simulink model "Xcvr_SSB_AM_2p5"  (Simulink 7.4)
settings: Solver=VariableStepDiscrete  SolverMode=SingleTasking  StartTime=0.0  StopTime=10  RelTol=1e-3
PreLoadFcn:
  | Fs=80e6;
  | 
  | phee=da_rom();
  | [phee_1,phee_2]=da_i2_rom();
  | 
  | Dcic=64;       % CIC decimation
  | Dfac=128;    % following DA filter decimation
  | N = 6;           %       (2^(N+1))=Dfac
  | Daudio=Dcic*Dfac;
  | Faudio=Fs/Daudio;
  | 
  | load info_filt_ssb_4
  | load Serial_Intfc_Stream_5
  | 
  | % AGC related
  | x=0.5:1/256:(1-1/256);
  | addr=(x-0.5)*256;
  | y=1./x;
undefined symbols (not defined in the file): Serial_Interface, ssb_coef, xlipgetpartsetting
libraries: xbsIndex_r4 x1305, dspsrcs4 x5, simulink x2, dspsigops x2, dspsnks4 x1
(part 8 of 11)

== system Xcvr_SSB_AM_2p5/TX Filters I=8192/Interp_Core/ROM/Accumulator ==
  Xn + Xn-4 : Inport
  "Xn-1+ Xn-3 " : Inport  Port=2
  Xn-2 : Inport  Port=3
  Yn-1 : Inport  Port=4
  Yn-2 : Inport  Port=5
  Xn+Xn-3 : Inport  Port=6
  Xn-1+Xn-2 : Inport  Port=7
  Zn-1 : Inport  Port=8
  Zn-2 : Inport  Port=9
  Round : Inport  Port=10
  Clear Acc : Inport  Port=11
  Subtract : Inport  Port=12
  AddSub{,1..3} (4 alike) : xbsIndex_r4/AddSub  mode=Addition  use_carryin=off  use_carryout=off  en=off  latency=0  precision=User Defined  arith_type="Signed  (2's comp)"  n_bits=18+1  bin_pt=0  quantization=Truncate  overflow=Wrap  dbl_ovrd=off  use_behavioral_HDL=off  hw_selection=Fabric  pipelined=off  use_rpm=on  block_type=addsub
      settings: block_version=9.2.00
  Concat : xbsIndex_r4/Concat  num_inputs=6  dbl_ovrd=off  block_type=concat
      settings: block_version=9.2.00
  Concat1 : xbsIndex_r4/Concat  num_inputs=5  dbl_ovrd=off  block_type=concat
      settings: block_version=9.2.00
  Convert : xbsIndex_r4/Convert  arith_type="Signed  (2's comp)"  n_bits=2  bin_pt=0  quantization=Truncate  overflow=Wrap  en=off  latency=0  dbl_ovrd=off  pipeline=off  block_type=convert
      settings: block_version=9.2.00
  Phee_1 ROM : xbsIndex_r4/ROM  depth=64  initVector=phee_1  distributed_mem=Block RAM  rst=off  init_reg=0  en=off  latency=1  arith_type="Signed  (2's comp)"  n_bits=13  bin_pt=0  dbl_ovrd=off  optimize=Area  use_rpm=on  block_type=sprom
      settings: block_version=9.2.00
  Phee_2 ROM : xbsIndex_r4/ROM  depth=32  initVector=phee_2  distributed_mem=Block RAM  rst=off  init_reg=0  en=off  latency=1  arith_type="Signed  (2's comp)"  n_bits=13  bin_pt=0  dbl_ovrd=off  optimize=Area  use_rpm=on  block_type=sprom
      settings: block_version=9.2.00
  Register1 : xbsIndex_r4/Register  init=0  rst=on  en=off  dbl_ovrd=off  block_type=register
      settings: block_version=9.2.00
  Register2 : xbsIndex_r4/Register  init=0  rst=on  en=off  dbl_ovrd=off  block_type=register
      settings: block_version=9.2.00
  Reinterpret1 : xbsIndex_r4/Reinterpret  force_arith_type=on  arith_type="Signed  (2's comp)"  force_bin_pt=on  bin_pt=0  block_type=reinterpret
      settings: infoedit="Changes signal type without altering the binary representation.   You can changed the signal between signed and unsigned, and relocate the binary point.<P><P>Hardware notes: In hardware this block costs nothing.<P><P>Example:  Suppose the input is 6 bits wide, signed, with 2 fractional bits, and the output is forced to unsigned with 0 fractional bits.  Then an input of -2.0 (1110.00 in binary 2's complement) becomes an output of 56 (111000 in binary)."  block_version=9.2.00
  Reinterpret2 : xbsIndex_r4/Reinterpret  force_arith_type=on  arith_type="Signed  (2's comp)"  force_bin_pt=on  bin_pt=0  block_type=reinterpret
      settings: infoedit="Changes signal type without altering the binary representation.   You can changed the signal between signed and unsigned, and relocate the binary point.<P><P>Hardware notes: In hardware this block costs nothing.<P><P>Example:  Suppose the input is 6 bits wide, signed, with 2 fractional bits, and the output is forced to unsigned with 0 fractional bits.  Then an input of -2.0 (1110.00 in binary 2's complement) becomes an output of 56 (111000 in binary)."  block_version=9.2.00
  Shift1 : xbsIndex_r4/Shift  shift_dir=Left  shift_bits=5  en=off  latency=0  precision=User Defined  arith_type="Signed  (2's comp)"  n_bits=18  bin_pt=0  quantization=Truncate  overflow=Wrap  dbl_ovrd=off  block_type=shift
      settings: block_version=9.2.00
  Shift2 : xbsIndex_r4/Shift  shift_dir=Left  shift_bits=5  en=off  latency=0  precision=User Defined  arith_type="Signed  (2's comp)"  n_bits=18  bin_pt=0  quantization=Truncate  overflow=Wrap  dbl_ovrd=off  block_type=shift
      settings: block_version=9.2.00
  Shift3 : xbsIndex_r4/Shift  shift_dir=Right  shift_bits=1  en=off  latency=0  precision=Full  arith_type="Signed  (2's comp)"  n_bits=18  bin_pt=0  quantization=Truncate  overflow=Wrap  dbl_ovrd=off  block_type=shift
      settings: block_version=9.2.00
  Shift4 : xbsIndex_r4/Shift  shift_dir=Right  shift_bits=1  en=off  latency=0  precision=Full  arith_type="Signed  (2's comp)"  n_bits=18  bin_pt=0  quantization=Truncate  overflow=Wrap  dbl_ovrd=off  block_type=shift
      settings: block_version=9.2.00
  Slice1 : xbsIndex_r4/Slice  nbits=16  boolean_output=off  mode=Lower Bit Location + Width  bit1=0  base1=MSB of Input  bit0=0  base0=LSB of Input  dbl_ovrd=off  block_type=slice
      settings: infoedit="Extracts a given range of bits from each input sample and presents it at the output.  The output type is ordinarily unsigned with binary point at zero, but can be Boolean when the slice is one bit wide.<P><P>Hardware notes: In hardware this block costs nothing."  block_version=9.2.00
  Slice2 : xbsIndex_r4/Slice  nbits=16  boolean_output=off  mode=Lower Bit Location + Width  bit1=0  base1=MSB of Input  bit0=0  base0=LSB of Input  dbl_ovrd=off  block_type=slice
      settings: infoedit="Extracts a given range of bits from each input sample and presents it at the output.  The output type is ordinarily unsigned with binary point at zero, but can be Boolean when the slice is one bit wide.<P><P>Hardware notes: In hardware this block costs nothing."  block_version=9.2.00
  Yn : Outport
  Zn : Outport  Port=2
  wires:
  Round/1 -> Convert/1  "Round"
  Phee_1 ROM/1 -> Shift1/1
  Reinterpret1/1 -> Yn/1
  Concat/1 -> Phee_1 ROM/1
  Xn + Xn-4/1 -> Concat/6
  "Xn-1+ Xn-3 "/1 -> Concat/5
  Xn-2/1 -> Concat/4
  Yn-1/1 -> Concat/3
  Yn-2/1 -> Concat/2
  Phee_2 ROM/1 -> Shift2/1
  Reinterpret2/1 -> Zn/1
  Xn+Xn-3/1 -> Concat1/5
  Xn-1+Xn-2/1 -> Concat1/4
  Zn-1/1 -> Concat1/3
  Zn-2/1 -> Concat1/2
  Subtract/1 -> Concat/1, Concat1/1
  Convert/1 -> AddSub1/2, AddSub2/2
  Concat1/1 -> Phee_2 ROM/1
  Shift1/1 -> AddSub1/1
  Shift2/1 -> AddSub2/1
  AddSub1/1 -> AddSub/2
  AddSub2/1 -> AddSub3/2
  AddSub/1 -> Register2/1
  Register2/1 -> Slice2/1, Shift3/1
  AddSub3/1 -> Register1/1
  Register1/1 -> Slice1/1, Shift4/1
  Clear Acc/1 -> Register2/2, Register1/2  "Reset"
  Slice1/1 -> Reinterpret2/1
  Slice2/1 -> Reinterpret1/1
  Shift3/1 -> AddSub/1
  Shift4/1 -> AddSub3/1

== system Xcvr_SSB_AM_2p5/TX Filters I=8192/Interp_Core/SAD_1 ==
  A : Inport
  B : Inport  Port=2
  Clear : Inport  Port=3
  Full Adder : Subsystem
  Register : xbsIndex_r4/Register  init=0  rst=on  en=off  dbl_ovrd=off  block_type=register
      settings: block_version=9.2.00
  Sum : Outport
  wires:
  Clear/1 -> Register/2
  B/1 -> Full Adder/2(B)
  Full Adder/1(Sum) -> Sum/1
  A/1 -> Full Adder/1(A)
  Register/1 -> Full Adder/3(Cin)
  Full Adder/2(Cout) -> Register/1

== system Xcvr_SSB_AM_2p5/TX Filters I=8192/Interp_Core/SAD_2 ==
  A : Inport
  B : Inport  Port=2
  Clear : Inport  Port=3
  Full Adder : Subsystem
  Register : xbsIndex_r4/Register  init=0  rst=on  en=off  dbl_ovrd=off  block_type=register
      settings: block_version=9.2.00
  Sum : Outport
  wires:
  Full Adder/2(Cout) -> Register/1
  Register/1 -> Full Adder/3(Cin)
  A/1 -> Full Adder/1(A)
  Full Adder/1(Sum) -> Sum/1
  B/1 -> Full Adder/2(B)
  Clear/1 -> Register/2

== system Xcvr_SSB_AM_2p5/TX Filters I=8192/Interp_Core/SAD_3 ==
  A : Inport
  B : Inport  Port=2
  Clear : Inport  Port=3
  Full Adder : Subsystem
  Register : xbsIndex_r4/Register  init=0  rst=on  en=off  dbl_ovrd=off  block_type=register
      settings: block_version=9.2.00
  Sum : Outport
  wires:
  Clear/1 -> Register/2
  B/1 -> Full Adder/2(B)
  Full Adder/1(Sum) -> Sum/1
  A/1 -> Full Adder/1(A)
  Register/1 -> Full Adder/3(Cin)
  Full Adder/2(Cout) -> Register/1

== system Xcvr_SSB_AM_2p5/TX Filters I=8192/Interp_Core/SAD_4 ==
  A : Inport
  B : Inport  Port=2
  Clear : Inport  Port=3
  Full Adder : Subsystem
  Register : xbsIndex_r4/Register  init=0  rst=on  en=off  dbl_ovrd=off  block_type=register
      settings: block_version=9.2.00
  Sum : Outport
  wires:
  Full Adder/2(Cout) -> Register/1
  Register/1 -> Full Adder/3(Cin)
  A/1 -> Full Adder/1(A)
  Full Adder/1(Sum) -> Sum/1
  B/1 -> Full Adder/2(B)
  Clear/1 -> Register/2

== system Xcvr_SSB_AM_2p5/TX Filters I=8192/Interp_Core/SRA ==
  Par_In : Inport
  Shift : Inport  Port=2
  Delay : xbsIndex_r4/Delay  en=off  latency=1  dbl_ovrd=off  reg_retiming=off  block_type=delay
      settings: block_version=9.2.00
  Delay1 : xbsIndex_r4/Delay  en=off  latency=1  dbl_ovrd=off  reg_retiming=off  block_type=delay
      settings: block_version=9.2.00
  Mux : xbsIndex_r4/Mux  inputs=2  en=off  latency=0  precision=Full  arith_type=Unsigned  n_bits=16  bin_pt=14  quantization=Truncate  overflow=Wrap  dbl_ovrd=off  block_type=mux
      settings: block_version=9.2.00
  Shift1 : xbsIndex_r4/Shift  shift_dir=Right  shift_bits=1  en=off  latency=0  precision=Full  arith_type="Signed  (2's comp)"  n_bits=16  bin_pt=14  quantization=Truncate  overflow=Wrap  dbl_ovrd=off  block_type=shift
      settings: block_version=9.2.00
  Slice : xbsIndex_r4/Slice  nbits=1  boolean_output=on  mode=Lower Bit Location + Width  bit1=0  base1=MSB of Input  bit0=0  base0=LSB of Input  dbl_ovrd=off  block_type=slice
      settings: infoedit="Extracts a given range of bits from each input sample and presents it at the output.  The output type is ordinarily unsigned with binary point at zero, but can be Boolean when the slice is one bit wide.<P><P>Hardware notes: In hardware this block costs nothing."  block_version=9.2.00
  Ser_Out : Outport
  wires:
  Delay1/1 -> Ser_Out/1
  Par_In/1 -> Mux/2
  Shift/1 -> Mux/1
  Shift1/1 -> Delay/1
  Slice/1 -> Delay1/1
  Delay/1 -> Mux/3
  Mux/1 -> Shift1/1, Slice/1

== system Xcvr_SSB_AM_2p5/TX Filters I=8192/Interp_Core/SR_Yn ==
  Par_In : Inport
  Shift : Inport  Port=2
  Delay : xbsIndex_r4/Delay  en=off  latency=1  dbl_ovrd=off  reg_retiming=off  block_type=delay
      settings: block_version=9.2.00
  Delay1 : xbsIndex_r4/Delay  en=off  latency=1  dbl_ovrd=off  reg_retiming=off  block_type=delay
      settings: block_version=9.2.00
  Mux : xbsIndex_r4/Mux  inputs=2  en=off  latency=0  precision=Full  arith_type=Unsigned  n_bits=16  bin_pt=14  quantization=Truncate  overflow=Wrap  dbl_ovrd=off  block_type=mux
      settings: block_version=9.2.00
  Shift1 : xbsIndex_r4/Shift  shift_dir=Right  shift_bits=1  en=off  latency=0  precision=Full  arith_type="Signed  (2's comp)"  n_bits=16  bin_pt=14  quantization=Truncate  overflow=Wrap  dbl_ovrd=off  block_type=shift
      settings: block_version=9.2.00
  Slice : xbsIndex_r4/Slice  nbits=1  boolean_output=on  mode=Lower Bit Location + Width  bit1=0  base1=MSB of Input  bit0=0  base0=LSB of Input  dbl_ovrd=off  block_type=slice
      settings: infoedit="Extracts a given range of bits from each input sample and presents it at the output.  The output type is ordinarily unsigned with binary point at zero, but can be Boolean when the slice is one bit wide.<P><P>Hardware notes: In hardware this block costs nothing."  block_version=9.2.00
  Ser_Out : Outport
  wires:
  Mux/1 -> Slice/1, Shift1/1
  Delay/1 -> Mux/3
  Slice/1 -> Delay1/1
  Shift1/1 -> Delay/1
  Shift/1 -> Mux/1
  Par_In/1 -> Mux/2
  Delay1/1 -> Ser_Out/1

== system Xcvr_SSB_AM_2p5/TX Filters I=8192/Interp_Core/SR_Zn ==
  Par_In : Inport
  Shift : Inport  Port=2
  Delay : xbsIndex_r4/Delay  en=off  latency=1  dbl_ovrd=off  reg_retiming=off  block_type=delay
      settings: block_version=9.2.00
  Delay1 : xbsIndex_r4/Delay  en=off  latency=1  dbl_ovrd=off  reg_retiming=off  block_type=delay
      settings: block_version=9.2.00
  Mux : xbsIndex_r4/Mux  inputs=2  en=off  latency=0  precision=Full  arith_type=Unsigned  n_bits=16  bin_pt=14  quantization=Truncate  overflow=Wrap  dbl_ovrd=off  block_type=mux
      settings: block_version=9.2.00
  Shift1 : xbsIndex_r4/Shift  shift_dir=Right  shift_bits=1  en=off  latency=0  precision=Full  arith_type="Signed  (2's comp)"  n_bits=16  bin_pt=14  quantization=Truncate  overflow=Wrap  dbl_ovrd=off  block_type=shift
      settings: block_version=9.2.00
  Slice : xbsIndex_r4/Slice  nbits=1  boolean_output=on  mode=Lower Bit Location + Width  bit1=0  base1=MSB of Input  bit0=0  base0=LSB of Input  dbl_ovrd=off  block_type=slice
      settings: infoedit="Extracts a given range of bits from each input sample and presents it at the output.  The output type is ordinarily unsigned with binary point at zero, but can be Boolean when the slice is one bit wide.<P><P>Hardware notes: In hardware this block costs nothing."  block_version=9.2.00
  Ser_Out : Outport
  wires:
  Delay1/1 -> Ser_Out/1
  Par_In/1 -> Mux/2
  Shift/1 -> Mux/1
  Shift1/1 -> Delay/1
  Slice/1 -> Delay1/1
  Delay/1 -> Mux/3
  Mux/1 -> Shift1/1, Slice/1

== system Xcvr_SSB_AM_2p5/TX Filters I=8192/Interp_Core/Timing/Control1 ==
  Start : Inport
  AddSub : xbsIndex_r4/AddSub  mode=Addition  use_carryin=off  use_carryout=off  en=off  latency=0  precision=User Defined  arith_type=Unsigned  n_bits=5  bin_pt=0  quantization=Truncate  overflow=Wrap  dbl_ovrd=off  use_behavioral_HDL=off  hw_selection=Fabric  pipelined=off  use_rpm=on  block_type=addsub
      settings: block_version=9.2.00
  Constant : xbsIndex_r4/Constant  arith_type=Unsigned  const=21  n_bits=5  bin_pt=0  explicit_period=off  period=1  equ=P=C  opselect=C  inp2=PCIN>>17  opr=+  inp1=P  carry=CIN  dbl_ovrd=off  block_type=constant
      settings: block_version=9.2.00
  Constant1 : xbsIndex_r4/Constant  arith_type=Unsigned  const=1  n_bits=5  bin_pt=0  explicit_period=off  period=1  equ=P=C  opselect=C  inp2=PCIN>>17  opr=+  inp1=P  carry=CIN  dbl_ovrd=off  block_type=constant
      settings: block_version=9.2.00
  Constant10 : xbsIndex_r4/Constant  arith_type=Unsigned  const=17  n_bits=5  bin_pt=0  explicit_period=off  period=1  equ=P=C  opselect=C  inp2=PCIN>>17  opr=+  inp1=P  carry=CIN  dbl_ovrd=off  block_type=constant
      settings: block_version=9.2.00
  Constant12 : xbsIndex_r4/Constant  arith_type=Unsigned  const=2  n_bits=5  bin_pt=0  explicit_period=off  period=1  equ=P=C  opselect=C  inp2=PCIN>>17  opr=+  inp1=P  carry=CIN  dbl_ovrd=off  block_type=constant
      settings: block_version=9.2.00
  Constant2 : xbsIndex_r4/Constant  arith_type=Unsigned  const=0  n_bits=5  bin_pt=0  explicit_period=off  period=1  equ=P=C  opselect=C  inp2=PCIN>>17  opr=+  inp1=P  carry=CIN  dbl_ovrd=off  block_type=constant
      settings: block_version=9.2.00
  Constant3 : xbsIndex_r4/Constant  arith_type=Unsigned  const=0  n_bits=5  bin_pt=0  explicit_period=off  period=1  equ=P=C  opselect=C  inp2=PCIN>>17  opr=+  inp1=P  carry=CIN  dbl_ovrd=off  block_type=constant
      settings: block_version=9.2.00
  Constant4 : xbsIndex_r4/Constant  arith_type=Unsigned  const=1  n_bits=5  bin_pt=0  explicit_period=off  period=1  equ=P=C  opselect=C  inp2=PCIN>>17  opr=+  inp1=P  carry=CIN  dbl_ovrd=off  block_type=constant
      settings: block_version=9.2.00
  Constant5 : xbsIndex_r4/Constant  arith_type=Unsigned  const=20  n_bits=5  bin_pt=0  explicit_period=off  period=1  equ=P=C  opselect=C  inp2=PCIN>>17  opr=+  inp1=P  carry=CIN  dbl_ovrd=off  block_type=constant
      settings: block_version=9.2.00
  Constant6 : xbsIndex_r4/Constant  arith_type=Unsigned  const=18  n_bits=5  bin_pt=0  explicit_period=off  period=1  equ=P=C  opselect=C  inp2=PCIN>>17  opr=+  inp1=P  carry=CIN  dbl_ovrd=off  block_type=constant
      settings: block_version=9.2.00
  Constant7 : xbsIndex_r4/Constant  arith_type=Unsigned  const=2-1  n_bits=5  bin_pt=0  explicit_period=off  period=1  equ=P=C  opselect=C  inp2=PCIN>>17  opr=+  inp1=P  carry=CIN  dbl_ovrd=off  block_type=constant
      settings: block_version=9.2.00
  Constant8 : xbsIndex_r4/Constant  arith_type=Unsigned  const=17-1  n_bits=5  bin_pt=0  explicit_period=off  period=1  equ=P=C  opselect=C  inp2=PCIN>>17  opr=+  inp1=P  carry=CIN  dbl_ovrd=off  block_type=constant
      settings: block_version=9.2.00
  Constant9 : xbsIndex_r4/Constant  arith_type=Unsigned  const=18  n_bits=5  bin_pt=0  explicit_period=off  period=1  equ=P=C  opselect=C  inp2=PCIN>>17  opr=+  inp1=P  carry=CIN  dbl_ovrd=off  block_type=constant
      settings: block_version=9.2.00
  Delay : xbsIndex_r4/Delay  en=off  latency=1  dbl_ovrd=off  reg_retiming=off  block_type=delay
      settings: block_version=9.2.00
  Logical : xbsIndex_r4/Logical  logical_function=AND  inputs=2  en=off  latency=0  precision=Full  arith_type=Unsigned  n_bits=16  bin_pt=0  align_bp=on  dbl_ovrd=off  block_type=logical
      settings: block_version=9.2.00
  Mux : xbsIndex_r4/Mux  inputs=2  en=off  latency=0  precision=Full  arith_type=Unsigned  n_bits=16  bin_pt=14  quantization=Truncate  overflow=Wrap  dbl_ovrd=off  block_type=mux
      settings: block_version=9.2.00
  Relational{,2..4,7..8,10} (7 alike) : xbsIndex_r4/Relational  mode=a=b  en=off  latency=0  dbl_ovrd=off  block_type=relational
      settings: block_version=9.2.00
  Relational1 : xbsIndex_r4/Relational  mode=a>b  en=off  latency=0  dbl_ovrd=off  block_type=relational
      settings: block_version=9.2.00
  Relational5 : xbsIndex_r4/Relational  mode=a>=b  en=off  latency=0  dbl_ovrd=off  block_type=relational
      settings: block_version=9.2.00
  Relational6 : xbsIndex_r4/Relational  mode=a<=b  en=off  latency=0  dbl_ovrd=off  block_type=relational
      settings: block_version=9.2.00
  S-R FF1 : Subsystem
  SR Enable : Outport
  Run : Outport  Port=2
  Clear_Adder : Outport  Port=3
  Round : Outport  Port=4
  Clear_Acc : Outport  Port=5
  Subtract : Outport  Port=6
  Strobe : Outport  Port=7
  Valid : Outport  Port=8
  Extend_Sign : Outport  Port=9
  wires:
  Relational4/1 -> Subtract/1
  Relational1/1 -> Run/1
  Delay/1 -> Relational5/1, Relational6/1, Relational7/1, Relational8/1, Relational3/1, Relational2/1, AddSub/1, Relational/1, Relational1/1, Relational10/1, Relational4/1
  Relational/1 -> S-R FF1/2(Reset), Valid/1
  Constant/1 -> Relational/2
  S-R FF1/1(Q) -> Mux/1
  Start/1 -> S-R FF1/1(Set)
  Mux/1 -> Delay/1
  AddSub/1 -> Mux/3
  Constant1/1 -> AddSub/2
  Constant2/1 -> Mux/2
  Constant3/1 -> Relational1/2
  Constant4/1 -> Relational2/2
  Relational2/1 -> Clear_Adder/1
  Constant5/1 -> Relational3/2
  Relational3/1 -> Strobe/1
  Constant6/1 -> Relational4/2
  Constant7/1 -> Relational5/2
  Constant8/1 -> Relational6/2
  Relational5/1 -> Logical/1
  Relational6/1 -> Logical/2
  Logical/1 -> SR Enable/1
  Constant9/1 -> Relational7/2
  Relational7/1 -> Round/1
  Constant12/1 -> Relational10/2
  Relational10/1 -> Clear_Acc/1
  Constant10/1 -> Relational8/2
  Relational8/1 -> Extend_Sign/1

== system Xcvr_SSB_AM_2p5/Up/Down LO and Mixers/Delay allow T/R  Relay time./N_Sample_One_Shot ==
  In : Inport  OutDataType=fixdt(1, 16)  OutScaling=2^0
  Counter : xbsIndex_r4/Counter  cnt_type=Free Running  cnt_to=Inf  operation=Up  start_count=0  cnt_by_val=1  arith_type=Unsigned  n_bits=8  bin_pt=0  load_pin=off  rst=on  en=off  explicit_period=off  period=1  dbl_ovrd=off  use_behavioral_HDL=off  implementation=Fabric  block_type=counter
      settings: block_version=12.1
  Inverter : xbsIndex_r4/Inverter  en=off  latency=0  dbl_ovrd=off  block_type=inv
      settings: block_version=12.1
  Logical : xbsIndex_r4/Logical  logical_function=OR  inputs=2  en=off  latency=0  precision=Full  arith_type=Unsigned  n_bits=16  bin_pt=0  align_bp=on  dbl_ovrd=off  block_type=logical
      settings: block_version=12.1
  N : xbsIndex_r4/Constant  arith_type=Unsigned  const=N  n_bits=8  bin_pt=0  explicit_period=off  period=1  equ=P=C  opselect=C  inp2=PCIN>>17  opr=+  inp1=P  carry=CIN  dbl_ovrd=off  block_type=constant
      settings: block_version=12.1
  Register : xbsIndex_r4/Register  init=0  rst=on  en=off  dbl_ovrd=off  block_type=register
      settings: block_version=12.1
  Relational : xbsIndex_r4/Relational  mode=a=b  en=off  latency=0  dbl_ovrd=off  block_type=relational
      settings: block_version=12.1
  Out : Outport  OutDataType=fixdt(1, 16)  OutScaling=2^0
  wires:
  Logical/1 -> Register/1, Out/1
  Register/1 -> Logical/2, Inverter/1
  In/1 -> Logical/1
  Counter/1 -> Relational/1
  N/1 -> Relational/2
  Relational/1 -> Register/2
  Inverter/1 -> Counter/1

== system Xcvr_SSB_AM_2p5/Audio_and_Mode_Control/AGC_and_More/AGC Xilinx/AGC_Reg ==
  note: This circuit ensures that the RX AGC Divisor is never 0.
  note: Bits 15 - 0 (16):  fixed RX Gain
      | Bits 17-16 (2):  fixed TX Gain
      | Bits 22-18 (5): Hang Time
      | Bit 23-24 (2):  Decay Rate
      | Bit25:  k6jca/w1qg AGC Select
  WR_AGC : Inport  OutDataType=fixdt(1, 16)  OutScaling=2^0
  Data_in : Inport  Port=2  OutDataType=fixdt(1, 16)  OutScaling=2^0
  AGC_Decay_b23 : xbsIndex_r4/Slice  nbits=2  boolean_output=off  mode=Lower Bit Location + Width  bit1=-2  base1=MSB of Input  bit0=23  base0=LSB of Input  dbl_ovrd=off  block_type=slice
      settings: block_version=9.2.00
  AGC_Decay_b25 : xbsIndex_r4/Slice  nbits=1  boolean_output=on  mode=Lower Bit Location + Width  bit1=-2  base1=MSB of Input  bit0=25  base0=LSB of Input  dbl_ovrd=off  block_type=slice
      settings: block_version=9.2.00
  AGC_Hang_b18 : xbsIndex_r4/Slice  nbits=5  boolean_output=off  mode=Lower Bit Location + Width  bit1=-2  base1=MSB of Input  bit0=18  base0=LSB of Input  dbl_ovrd=off  block_type=slice
      settings: block_version=9.2.00
  Constant2 : xbsIndex_r4/Constant  arith_type=Unsigned  const=0  n_bits=16  bin_pt=0  explicit_period=off  period=1  equ=P=C  opselect=C  inp2=PCIN>>17  opr=+  inp1=P  carry=CIN  dbl_ovrd=off  block_type=constant
      settings: block_version=12.1
  Constant4 : xbsIndex_r4/Constant  arith_type=Unsigned  const=1  n_bits=16  bin_pt=0  explicit_period=off  period=1  equ=P=C  opselect=C  inp2=PCIN>>17  opr=+  inp1=P  carry=CIN  dbl_ovrd=off  block_type=constant
      settings: block_version=12.1
  Down Sample1 : xbsIndex_r4/Down Sample  sample_ratio=1024  sample_phase="Last Value of Frame  (most efficient)"  en=off  latency=1  dbl_ovrd=off  block_type=dsamp
      settings: block_version=9.2.00
  Mux3 : xbsIndex_r4/Mux  inputs=2  en=off  latency=0  precision=Full  arith_type=Unsigned  n_bits=26  bin_pt=26  quantization=Truncate  overflow=Wrap  dbl_ovrd=off  block_type=mux
      settings: block_version=9.2.00
  Register1 : xbsIndex_r4/Register  init=0  rst=off  en=on  dbl_ovrd=off  block_type=register
      settings: block_version=9.2.00
  Reinterpret1 : xbsIndex_r4/Reinterpret  force_arith_type=on  arith_type=Unsigned  force_bin_pt=on  bin_pt=16  block_type=reinterpret
      settings: infoedit="Changes signal type without altering the binary representation.   You can changed the signal between signed and unsigned, and relocate the binary point.<br><br>Hardware notes: In hardware this block costs nothing.<br><br>Example:  Suppose the input is 6 bits wide, signed, with 2 fractional bits, and the output is forced to unsigned with 0 fractional bits.  Then an input of -2.0 (1110.00 in binary 2's complement) becomes an output of 56 (111000 in binary)."  block_version=9.2.00
  Relational5 : xbsIndex_r4/Relational  mode=a=b  en=off  latency=0  dbl_ovrd=off  block_type=relational
      settings: block_version=9.2.00
  fixed_RX_gain : xbsIndex_r4/Slice  nbits=16  boolean_output=off  mode=Lower Bit Location + Width  bit1=-2  base1=MSB of Input  bit0=0  base0=LSB of Input  dbl_ovrd=off  block_type=slice
      settings: block_version=9.2.00
  fixed_TX_gain_b16 : xbsIndex_r4/Slice  nbits=2  boolean_output=off  mode=Lower Bit Location + Width  bit1=-2  base1=MSB of Input  bit0=16  base0=LSB of Input  dbl_ovrd=off  block_type=slice
      settings: block_version=9.2.00
  AGC_Hang : Outport  OutDataType=fixdt(1, 16)  OutScaling=2^0
  AGC_Decay_Rate : Outport  Port=2  OutDataType=fixdt(1, 16)  OutScaling=2^0
  Max_RX_Gain : Outport  Port=3  OutDataType=fixdt(1, 16)  OutScaling=2^0
  Max_Mic_Gain : Outport  Port=4  OutDataType=fixdt(1, 16)  OutScaling=2^0
  JCA_AGC : Outport  Port=5  OutDataType=fixdt(1, 16)  OutScaling=2^0
  wires:
  Down Sample1/1 -> fixed_RX_gain/1, fixed_TX_gain_b16/1, AGC_Hang_b18/1, AGC_Decay_b23/1, AGC_Decay_b25/1
  Register1/1 -> Down Sample1/1
  Relational5/1 -> Mux3/1
  Mux3/1 -> Reinterpret1/1
  Constant2/1 -> Relational5/1
  fixed_RX_gain/1 -> Relational5/2, Mux3/2
  Constant4/1 -> Mux3/3
  WR_AGC/1 -> Register1/2
  Data_in/1 -> Register1/1
  Reinterpret1/1 -> Max_RX_Gain/1
  fixed_TX_gain_b16/1 -> Max_Mic_Gain/1
  AGC_Hang_b18/1 -> AGC_Hang/1
  AGC_Decay_b23/1 -> AGC_Decay_Rate/1
  AGC_Decay_b25/1 -> JCA_AGC/1

== system Xcvr_SSB_AM_2p5/Audio_and_Mode_Control/AGC_and_More/AGC Xilinx/Attack Filter ==
  note: (6/32)/(1-(1-.0625)Z^-1)
  JCA_AGC : Inport
  Abs_In1 : Inport  Port=2
  Trans_Reset : Inport  Port=3
  AddSub : xbsIndex_r4/AddSub  mode=Addition  use_carryin=off  use_carryout=off  en=off  latency=0  precision=User Defined  arith_type=Unsigned  n_bits=24  bin_pt=20  quantization="Round  (unbiased: +/- Inf)"  overflow=Wrap  dbl_ovrd=off  use_behavioral_HDL=off  hw_selection=Fabric  pipelined=off  use_rpm=on  block_type=addsub
      settings: block_version=9.2.00
  CMult1 : xbsIndex_r4/CMult  const=6/32  const_n_bits=5  const_bin_pt=5  en=off  latency=0  precision=User Defined  arith_type=Unsigned  n_bits=16  bin_pt=15  quantization="Round  (unbiased: +/- Inf)"  overflow=Saturate  dbl_ovrd=off  use_behavioral_HDL=off  mem_type=Distributed RAM  pipeline=off  use_rpm=off  placement_style=Rectangular Shape  block_type=cmult
      settings: block_version=9.2.00
  CMult2 : xbsIndex_r4/CMult  const=(1-1/16)  const_n_bits=6  const_bin_pt=6  en=off  latency=0  precision=User Defined  arith_type=Unsigned  n_bits=24  bin_pt=20  quantization=Truncate  overflow=Saturate  dbl_ovrd=off  use_behavioral_HDL=off  mem_type=Distributed RAM  pipeline=off  use_rpm=off  placement_style=Rectangular Shape  block_type=cmult
      settings: block_version=9.2.00
  CMult3 : xbsIndex_r4/CMult  const=1.1875  const_n_bits=5  const_bin_pt=4  en=off  latency=0  precision=User Defined  arith_type=Unsigned  n_bits=16  bin_pt=15  quantization="Round  (unbiased: +/- Inf)"  overflow=Saturate  dbl_ovrd=off  use_behavioral_HDL=off  mem_type=Distributed RAM  pipeline=off  use_rpm=off  placement_style=Rectangular Shape  block_type=cmult
      settings: block_version=9.2.00
  Constant2 : xbsIndex_r4/Constant  arith_type=Unsigned  const=0  n_bits=24  bin_pt=20  explicit_period=off  period=1  equ=P=C  opselect=C  inp2=PCIN>>17  opr=+  inp1=P  carry=CIN  dbl_ovrd=off  block_type=constant
      settings: block_version=12.1
  Mux1 : xbsIndex_r4/Mux  inputs=2  en=off  latency=0  precision=User Defined  arith_type=Unsigned  n_bits=16  bin_pt=15  quantization=Truncate  overflow=Saturate  dbl_ovrd=off  block_type=mux
      settings: block_version=9.2.00
  Mux2 : xbsIndex_r4/Mux  inputs=2  en=off  latency=0  precision=Full  arith_type=Unsigned  n_bits=26  bin_pt=26  quantization=Truncate  overflow=Wrap  dbl_ovrd=off  block_type=mux
      settings: block_version=9.2.00
  Register1 : xbsIndex_r4/Register  init=0  rst=on  en=off  dbl_ovrd=off  block_type=register
      settings: block_version=9.2.00
  Out1 : Outport
  wires:
  AddSub/1 -> Register1/1
  Register1/1 -> CMult1/1, CMult3/1, CMult2/1
  Abs_In1/1 -> AddSub/1
  JCA_AGC/1 -> Mux1/1, Mux2/1
  CMult1/1 -> Mux1/2
  Mux1/1 -> Out1/1
  CMult3/1 -> Mux1/3
  Mux2/1 -> AddSub/2
  CMult2/1 -> Mux2/2
  Constant2/1 -> Mux2/3
  Trans_Reset/1 -> Register1/2

== system Xcvr_SSB_AM_2p5/Audio_and_Mode_Control/AGC_and_More/AGC Xilinx/Hang_Time ==
  note: While HANGING (Not_Hanging = 0), do not decay the AGC Value
  note: Force HANG to end if change between XMIT and RCV.
  note: Hangtime = Hang_load * 512 / (9765.625Hz)
      | (Increments of 52.4 ms)
  Tx_Rx_Delayed : Inport
  Hang_load : Inport  Port=2
  New_Max : Inport  Port=3
  Concat : xbsIndex_r4/Concat  num_inputs=2  dbl_ovrd=off  block_type=concat
      settings: block_version=12.1
  Constant1 : xbsIndex_r4/Constant  arith_type=Unsigned  const=0  n_bits=9  bin_pt=0  explicit_period=off  period=1  equ=P=C  opselect=C  inp2=PCIN>>17  opr=+  inp1=P  carry=CIN  dbl_ovrd=off  block_type=constant
      settings: block_version=12.1
  Constant2 : xbsIndex_r4/Constant  arith_type=Unsigned  const=0  n_bits=13  bin_pt=0  explicit_period=off  period=1  equ=P=C  opselect=C  inp2=PCIN>>17  opr=+  inp1=P  carry=CIN  dbl_ovrd=off  block_type=constant
      settings: block_version=12.1
  Counter : xbsIndex_r4/Counter  cnt_type=Free Running  cnt_to=0  operation=Down  start_count=0  cnt_by_val=1  arith_type=Unsigned  n_bits=14  bin_pt=0  load_pin=on  rst=on  en=on  explicit_period=off  period=1/Faudio  dbl_ovrd=off  use_behavioral_HDL=off  implementation=Fabric  block_type=counter
      settings: block_version=12.1
  Delay : xbsIndex_r4/Delay  en=off  latency=1  dbl_ovrd=off  reg_retiming=off  block_type=delay
      settings: block_version=9.2.00
  Inverter1 : xbsIndex_r4/Inverter  en=off  latency=0  dbl_ovrd=off  block_type=inv
      settings: block_version=9.2.00
  Logical2 : xbsIndex_r4/Logical  logical_function=XOR  inputs=2  en=off  latency=0  precision=Full  arith_type=Unsigned  n_bits=16  bin_pt=0  align_bp=on  dbl_ovrd=off  block_type=logical
      settings: block_version=12.1
  Logical3 : xbsIndex_r4/Logical  logical_function=OR  inputs=3  en=off  latency=0  precision=Full  arith_type=Unsigned  n_bits=16  bin_pt=0  align_bp=on  dbl_ovrd=off  block_type=logical
      settings: block_version=12.1
  Logical4 : xbsIndex_r4/Logical  logical_function=OR  inputs=2  en=off  latency=0  precision=Full  arith_type=Unsigned  n_bits=16  bin_pt=0  align_bp=on  dbl_ovrd=off  block_type=logical
      settings: block_version=12.1
  Relational : xbsIndex_r4/Relational  mode=a=b  en=off  latency=0  dbl_ovrd=off  block_type=relational
      settings: block_version=9.2.00
  Trans_Reset : Outport
  Not_Hanging : Outport  Port=2
  Hang_TP : Outport  Port=3
  wires:
  New_Max/1 -> Logical4/1, Counter/1, Logical3/1
  Tx_Rx_Delayed/1 -> Delay/1, Logical2/1
  Delay/1 -> Logical2/2
  Logical2/1 -> Logical3/2, Counter/3, Trans_Reset/1
  Constant2/1 -> Relational/2
  Counter/1 -> Relational/1
  Relational/1 -> Inverter1/1, Logical4/2
  Inverter1/1 -> Logical3/3, Hang_TP/1
  Logical4/1 -> Not_Hanging/1
  Logical3/1 -> Counter/4
  Constant1/1 -> Concat/2
  Hang_load/1 -> Concat/1
  Concat/1 -> Counter/2

== system Xcvr_SSB_AM_2p5/Audio_and_Mode_Control/AGC_and_More/AGC Xilinx/Leaky Peak Detector ==
  note: Leaky Peak Detector
  Tx_Rx_Delayed : Inport  OutDataType=fixdt(1, 16)  OutScaling=2^0
  Rx_Tx_Delayed : Inport  Port=2  OutDataType=fixdt(1, 16)  OutScaling=2^0
  Abs_In2 : Inport  Port=3  OutDataType=fixdt(1, 16)  OutScaling=2^0
  En : Inport  Port=4  OutDataType=fixdt(1, 16)  OutScaling=2^0
  Rate : Inport  Port=5  OutDataType=fixdt(1, 16)  OutScaling=2^0
  Fast Decay : xbsIndex_r4/CMult  const=1-(2^-11)  const_n_bits=12  const_bin_pt=12  en=off  latency=0  precision=User Defined  arith_type=Unsigned  n_bits=24  bin_pt=23  quantization=Truncate  overflow=Wrap  dbl_ovrd=off  use_behavioral_HDL=off  mem_type=Distributed RAM  pipeline=off  use_rpm=off  placement_style=Rectangular Shape  block_type=cmult
      settings: block_version=9.2.00
  Logical1 : xbsIndex_r4/Logical  logical_function=AND  inputs=2  en=off  latency=0  precision=Full  arith_type=Unsigned  n_bits=16  bin_pt=0  align_bp=on  dbl_ovrd=off  block_type=logical
      settings: block_version=12.1
  Logical2 : xbsIndex_r4/Logical  logical_function=AND  inputs=2  en=off  latency=0  precision=Full  arith_type=Unsigned  n_bits=16  bin_pt=0  align_bp=on  dbl_ovrd=off  block_type=logical
      settings: block_version=12.1
  Mux : xbsIndex_r4/Mux  inputs=2  en=off  latency=0  precision=User Defined  arith_type=Unsigned  n_bits=24  bin_pt=23  quantization=Truncate  overflow=Wrap  dbl_ovrd=off  block_type=mux
      settings: block_version=9.2.00
  Mux1 : xbsIndex_r4/Mux  inputs=4  en=off  latency=0  precision=Full  arith_type=Unsigned  n_bits=16  bin_pt=16  quantization=Truncate  overflow=Wrap  dbl_ovrd=off  block_type=mux
      settings: block_version=9.2.00
  Mux2 : xbsIndex_r4/Mux  inputs=2  en=off  latency=0  precision=Full  arith_type=Unsigned  n_bits=26  bin_pt=26  quantization=Truncate  overflow=Wrap  dbl_ovrd=off  block_type=mux
      settings: block_version=9.2.00
  Register : xbsIndex_r4/Register  init=0  rst=off  en=on  dbl_ovrd=off  block_type=register
      settings: block_version=9.2.00
  Register1 : xbsIndex_r4/Register  init=0  rst=off  en=on  dbl_ovrd=off  block_type=register
      settings: block_version=9.2.00
  Relational : xbsIndex_r4/Relational  mode=a>b  en=off  latency=0  dbl_ovrd=off  block_type=relational
      settings: block_version=9.2.00
  Slow Decay : xbsIndex_r4/CMult  const=1-(2^-13)  const_n_bits=14  const_bin_pt=14  en=off  latency=0  precision=User Defined  arith_type=Unsigned  n_bits=24  bin_pt=23  quantization=Truncate  overflow=Wrap  dbl_ovrd=off  use_behavioral_HDL=off  mem_type=Distributed RAM  pipeline=off  use_rpm=off  placement_style=Rectangular Shape  block_type=cmult
      settings: block_version=9.2.00
  Very Fast : xbsIndex_r4/CMult  const=1-(2^-8)  const_n_bits=12  const_bin_pt=12  en=off  latency=0  precision=User Defined  arith_type=Unsigned  n_bits=24  bin_pt=23  quantization=Truncate  overflow=Wrap  dbl_ovrd=off  use_behavioral_HDL=off  mem_type=Distributed RAM  pipeline=off  use_rpm=off  placement_style=Rectangular Shape  block_type=cmult
      settings: block_version=9.2.00
  Very Very Fast : xbsIndex_r4/CMult  const=1-(2^-6)  const_n_bits=12  const_bin_pt=12  en=off  latency=0  precision=User Defined  arith_type=Unsigned  n_bits=24  bin_pt=23  quantization=Truncate  overflow=Wrap  dbl_ovrd=off  use_behavioral_HDL=off  mem_type=Distributed RAM  pipeline=off  use_rpm=off  placement_style=Rectangular Shape  block_type=cmult
      settings: block_version=9.2.00
  Out1 : Outport  OutDataType=fixdt(1, 16)  OutScaling=2^0
  New_Max : Outport  Port=2  OutDataType=fixdt(1, 16)  OutScaling=2^0
  wires:
  Abs_In2/1 -> Relational/1, Mux/3
  Relational/1 -> Mux/1, New_Max/1
  Fast Decay/1 -> Mux1/3
  Slow Decay/1 -> Mux1/2
  Mux1/1 -> Relational/2, Mux/2
  Mux/1 -> Register/1, Register1/1
  Register/1 -> Mux2/2
  Register1/1 -> Mux2/3
  Mux2/1 -> Slow Decay/1, Fast Decay/1, Very Very Fast/1, Very Fast/1, Out1/1
  Logical1/1 -> Register/2
  Logical2/1 -> Register1/2
  En/1 -> Logical2/2, Logical1/2
  Rx_Tx_Delayed/1 -> Logical1/1
  Tx_Rx_Delayed/1 -> Logical2/1, Mux2/1
  Rate/1 -> Mux1/1
  Very Fast/1 -> Mux1/4
  Very Very Fast/1 -> Mux1/5

== system Xcvr_SSB_AM_2p5/Audio_and_Mode_Control/AGC_and_More/AGC Xilinx/S-Meter ==
  note: TX Voice S-meter PWM
  note: TX CW S-meter PWM
  note: On  RX the S meter is log.
      | On TX the S Meter is linear.
  Tx_Rx_Delayed : Inport  OutDataType=fixdt(1, 16)  OutScaling=2^0
  RX_Smeter : Inport  Port=2  OutDataType=fixdt(1, 16)  OutScaling=2^0
  AGC_Divisor : Inport  Port=3  OutDataType=fixdt(1, 16)  OutScaling=2^0
  Tx_Rx : Inport  Port=4  OutDataType=fixdt(1, 16)  OutScaling=2^0
  CW_nSSB : Inport  Port=5  OutDataType=fixdt(1, 16)  OutScaling=2^0
  TX_Level : Inport  Port=6  OutDataType=fixdt(1, 16)  OutScaling=2^0
  Constant : xbsIndex_r4/Constant  arith_type=Unsigned  const=31  n_bits=5  bin_pt=0  explicit_period=off  period=1  equ=P=C  opselect=C  inp2=PCIN>>17  opr=+  inp1=P  carry=CIN  dbl_ovrd=off  block_type=constant
      settings: block_version=12.1
  Counter : xbsIndex_r4/Counter  cnt_type=Count Limited  cnt_to=31  operation=Up  start_count=0  cnt_by_val=1  arith_type=Unsigned  n_bits=5  bin_pt=0  load_pin=off  rst=off  en=off  explicit_period=on  period=1/(32*Faudio)  dbl_ovrd=off  use_behavioral_HDL=off  implementation=Fabric  use_rpm=off  block_type=counter
      settings: block_version=9.2.00
  Counter1 : xbsIndex_r4/Counter  cnt_type=Count Limited  cnt_to=31  operation=Up  start_count=0  cnt_by_val=1  arith_type=Unsigned  n_bits=5  bin_pt=0  load_pin=off  rst=off  en=off  explicit_period=on  period=1/(32*Faudio)  dbl_ovrd=off  use_behavioral_HDL=off  implementation=Fabric  use_rpm=off  block_type=counter
      settings: block_version=9.2.00
  Logical1 : xbsIndex_r4/Logical  logical_function=OR  inputs=2  en=off  latency=0  precision=Full  arith_type=Unsigned  n_bits=16  bin_pt=0  align_bp=on  dbl_ovrd=off  block_type=logical
      settings: block_version=12.1
  Logical3 : xbsIndex_r4/Logical  logical_function=AND  inputs=2  en=off  latency=0  precision=Full  arith_type=Unsigned  n_bits=16  bin_pt=0  align_bp=on  dbl_ovrd=off  block_type=logical
      settings: block_version=9.2.00
  Mux1 : xbsIndex_r4/Mux  inputs=2  en=off  latency=0  precision=Full  arith_type=Unsigned  n_bits=26  bin_pt=26  quantization=Truncate  overflow=Wrap  dbl_ovrd=off  block_type=mux
      settings: block_version=9.2.00
  Mux5 : xbsIndex_r4/Mux  inputs=2  en=off  latency=1  precision=Full  arith_type=Unsigned  n_bits=32  bin_pt=32  quantization="Round  (unbiased: +/- Inf)"  overflow=Wrap  dbl_ovrd=off  block_type=mux
      settings: block_version=9.2.00
  Mux6 : xbsIndex_r4/Mux  inputs=2  en=off  latency=0  precision=Full  arith_type=Unsigned  n_bits=26  bin_pt=26  quantization=Truncate  overflow=Wrap  dbl_ovrd=off  block_type=mux
      settings: block_version=9.2.00
  Relational1 : xbsIndex_r4/Relational  mode=a>b  en=off  latency=0  dbl_ovrd=off  block_type=relational
      settings: block_version=9.2.00
  Relational2 : xbsIndex_r4/Relational  mode=a>b  en=off  latency=0  dbl_ovrd=off  block_type=relational
      settings: block_version=9.2.00
  Slice1 : xbsIndex_r4/Slice  nbits=5  boolean_output=off  mode=Upper Bit Location + Width  bit1=-2  base1=MSB of Input  bit0=8  base0=LSB of Input  dbl_ovrd=off  block_type=slice
      settings: block_version=12.1
  Slice2 : xbsIndex_r4/Slice  nbits=1  boolean_output=on  mode=Upper Bit Location + Width  bit1=0  base1=MSB of Input  bit0=8  base0=LSB of Input  dbl_ovrd=off  block_type=slice
      settings: block_version=12.1
  Slice3 : xbsIndex_r4/Slice  nbits=1  boolean_output=on  mode=Upper Bit Location + Width  bit1=-1  base1=MSB of Input  bit0=8  base0=LSB of Input  dbl_ovrd=off  block_type=slice
      settings: block_version=12.1
  Slice4 : xbsIndex_r4/Slice  nbits=5  boolean_output=off  mode=Upper Bit Location + Width  bit1=0  base1=MSB of Input  bit0=8  base0=LSB of Input  dbl_ovrd=off  block_type=slice
      settings: block_version=12.1
  SMeter_PWM : Outport  OutDataType=fixdt(1, 16)  OutScaling=2^0
  wires:
  AGC_Divisor/1 -> Slice2/1, Slice3/1, Slice1/1
  Counter/1 -> Relational2/2
  Slice1/1 -> Mux1/2  "b18-b22"
  Mux1/1 -> Relational2/1
  Constant/1 -> Mux1/3
  Logical1/1 -> Mux1/1
  Slice2/1 -> Logical1/1  "b24"
  Slice3/1 -> Logical1/2  "b23"
  Tx_Rx_Delayed/1 -> Mux6/1
  RX_Smeter/1 -> Mux6/2
  Relational2/1 -> Mux6/3
  Counter1/1 -> Relational1/2
  Slice4/1 -> Relational1/1
  Relational1/1 -> Mux5/3
  Mux6/1 -> Mux5/2
  Mux5/1 -> SMeter_PWM/1
  Tx_Rx/1 -> Logical3/1
  CW_nSSB/1 -> Logical3/2
  Logical3/1 -> Mux5/1
  TX_Level/1 -> Slice4/1

== system Xcvr_SSB_AM_2p5/Audio_and_Mode_Control/AGC_and_More/AGC Xilinx/Sample Delay ==
  Sample_In : Inport  OutDataType=fixdt(1, 16)  OutScaling=2^0
  JCA_AGC : Inport  Port=2  OutDataType=fixdt(1, 16)  OutScaling=2^0
  Trans_Reset : Inport  Port=3  OutDataType=fixdt(1, 16)  OutScaling=2^0
  Mux3 : xbsIndex_r4/Mux  inputs=2  en=off  latency=0  precision=Full  arith_type=Unsigned  n_bits=24  bin_pt=23  quantization=Truncate  overflow=Wrap  dbl_ovrd=off  block_type=mux
      settings: block_version=9.2.00
  Register{,1..17} (18 alike) : xbsIndex_r4/Register  init=0  rst=on  en=off  dbl_ovrd=off  block_type=register
      settings: block_version=12.1
  Out1 : Outport  OutDataType=fixdt(1, 16)  OutScaling=2^0
  wires:
  Mux3/1 -> Out1/1
  Register/1 -> Register1/1
  Register1/1 -> Register2/1, Mux3/3
  Register2/1 -> Register3/1
  Register4/1 -> Register5/1
  Register6/1 -> Register7/1
  Register14/1 -> Register15/1
  Register13/1 -> Register14/1
  Register12/1 -> Register13/1
  Register11/1 -> Register12/1
  Register10/1 -> Register11/1
  Register9/1 -> Register10/1
  Register8/1 -> Register9/1
  Sample_In/1 -> Register/1
  JCA_AGC/1 -> Mux3/1
  Register3/1 -> Register4/1
  Register5/1 -> Register6/1
  Trans_Reset/1 -> Register8/2, Register14/2, Register15/2, Register17/2, Register13/2, Register12/2, Register11/2, Register10/2, Register9/2, Register6/2, Register7/2, Register16/2, Register5/2, Register4/2, Register3/2, Register2/2, Register1/2, Register/2
  Register7/1 -> Register16/1
  Register16/1 -> Register8/1
  Register17/1 -> Mux3/2
  Register15/1 -> Register17/1

== system Xcvr_SSB_AM_2p5/Audio_and_Mode_Control/AGC_and_More/AGC Xilinx/Sequential Divide ==
  note: Limit Max Tx or Rx Gain
  Tx_Rx_Delayed : Inport
  Dividend : Inport  Port=2
  Divisor : Inport  Port=3
  Max_RX_Gain : Inport  Port=4
  Max_Mic_Gain : Inport  Port=5
  AddSub : xbsIndex_r4/AddSub  mode=Addition  use_carryin=off  use_carryout=off  en=off  latency=0  precision=User Defined  arith_type=Unsigned  n_bits=16  bin_pt=16  quantization=Truncate  overflow=Saturate  dbl_ovrd=off  use_behavioral_HDL=off  hw_selection=Fabric  pipelined=off  use_rpm=on  block_type=addsub
      settings: block_version=9.2.00
  Constant1 : xbsIndex_r4/Constant  arith_type=Boolean  const=1  n_bits=16  bin_pt=16  explicit_period=off  period=1  equ=P=C  opselect=C  inp2=PCIN>>17  opr=+  inp1=P  carry=CIN  dbl_ovrd=off  block_type=constant
      settings: block_version=12.1
  Constant3 : xbsIndex_r4/Constant  arith_type=Unsigned  const=0  n_bits=16  bin_pt=16  explicit_period=off  period=1  equ=P=C  opselect=C  inp2=PCIN>>17  opr=+  inp1=P  carry=CIN  dbl_ovrd=off  block_type=constant
      settings: block_version=12.1
  Convert : xbsIndex_r4/Convert  arith_type=Unsigned  n_bits=4  bin_pt=0  quantization=Truncate  overflow=Wrap  en=off  latency=0  dbl_ovrd=off  pipeline=off  block_type=convert
      settings: block_version=9.2.00
  Convert1 : xbsIndex_r4/Convert  arith_type=Unsigned  n_bits=8  bin_pt=0  quantization=Truncate  overflow=Wrap  en=off  latency=0  dbl_ovrd=off  pipeline=off  block_type=convert
      settings: block_version=9.2.00
  Delay1 : xbsIndex_r4/Delay  en=off  latency=1  dbl_ovrd=off  reg_retiming=off  block_type=delay
      settings: block_version=9.2.00
  Down Sample : xbsIndex_r4/Down Sample  sample_ratio=32  sample_phase=First Value of Frame  en=off  latency=0  dbl_ovrd=off  block_type=dsamp
      settings: block_version=9.2.00
  Down Sample1 : xbsIndex_r4/Down Sample  sample_ratio=32  sample_phase=First Value of Frame  en=off  latency=0  dbl_ovrd=off  block_type=dsamp
      settings: block_version=9.2.00
  Gateway Out1 : xbsIndex_r4/Gateway Out  hdl_port=off  timing_constraint=None  locs_specified=off  LOCs={}  block_type=gatewayout
      settings: infoedit="Gateway out block.  Converts Xilinx fixed point inputs into ouputs of type Simulink integer, double, or fixed point.<br><br>Hardware notes:  In hardware these blocks become top level output ports or are discarded, depending on how they are configured."  block_version=12.1
  Mult : xbsIndex_r4/Mult  precision=User Defined  arith_type="Signed  (2's comp)"  n_bits=18  bin_pt=16  quantization=Truncate  overflow=Saturate  en=off  latency=0  dbl_ovrd=off  use_behavioral_HDL=off  opt=Speed  use_embedded=on  optimum_pipeline=off  pipeline=on  use_rpm=on  placement_style=Triangular  block_type=mult
      settings: block_version=9.2.00
  Mux1 : xbsIndex_r4/Mux  inputs=4  en=off  latency=0  precision=User Defined  arith_type=Unsigned  n_bits=16  bin_pt=16  quantization=Truncate  overflow=Wrap  dbl_ovrd=off  block_type=mux
      settings: block_version=9.2.00
  Mux5 : xbsIndex_r4/Mux  inputs=2  en=off  latency=0  precision=User Defined  arith_type=Unsigned  n_bits=16  bin_pt=16  quantization=Truncate  overflow=Wrap  dbl_ovrd=off  block_type=mux
      settings: block_version=9.2.00
  Mux6 : xbsIndex_r4/Mux  inputs=2  en=off  latency=0  precision=User Defined  arith_type=Unsigned  n_bits=16  bin_pt=16  quantization=Truncate  overflow=Wrap  dbl_ovrd=off  block_type=mux
      settings: block_version=9.2.00
  Relational1 : xbsIndex_r4/Relational  mode=a>b  en=off  latency=0  dbl_ovrd=off  block_type=relational
      settings: block_version=9.2.00
  Scale1 : xbsIndex_r4/Scale  scale_factor=-5  dbl_ovrd=off  block_type=scale
      settings: block_version=9.2.00
  Scale2 : xbsIndex_r4/Scale  scale_factor=-4  dbl_ovrd=off  block_type=scale
      settings: infoedit=Scales input by a power of two by adjusting the binary point position.<P><P>Hardware notes: In hardware this block costs nothing.  block_version=9.2.00
  Scale3 : xbsIndex_r4/Scale  scale_factor=-6  dbl_ovrd=off  block_type=scale
      settings: block_version=9.2.00
  Scale4 : xbsIndex_r4/Scale  scale_factor=-7  dbl_ovrd=off  block_type=scale
      settings: block_version=9.2.00
  Shift and lookup : Subsystem
  Up Sample : xbsIndex_r4/Up Sample  sample_ratio=32  copy_samples=on  en=off  latency=0  dbl_ovrd=off  block_type=usamp
      settings: block_version=9.2.00
  Up Sample1 : xbsIndex_r4/Up Sample  sample_ratio=32  copy_samples=on  en=off  latency=0  dbl_ovrd=off  block_type=usamp
      settings: block_version=9.2.00
  Variable Shifter : Subsystem  TreatAsAtomicUnit=on
  Audio : Outport
  Shift_TP : Outport  Port=2
  Smeter : Outport  Port=3
  tag scope: tpX=global
  wires:
  Delay1/1 -> Mult/2, Gateway Out1/1
  Shift and lookup/2(1/X) -> Mult/1
  Down Sample/1 -> Audio/1
  Variable Shifter/1(Out1) -> Down Sample/1
  Mult/1 -> Variable Shifter/2(Din)
  Up Sample/1 -> Delay1/1
  Shift and lookup/3(Shift) -> Convert/1, Down Sample1/1
  Shift and lookup/1(Ready) -> Variable Shifter/1(EN)
  Dividend/1 -> Up Sample/1
  Down Sample1/1 -> Shift_TP/1
  Shift and lookup/4(Smeter) -> Smeter/1
  Convert/1 -> Variable Shifter/3(Shift in)
  Gateway Out1/1 -> [tpX]
  Mux5/1 -> Relational1/1, Mux6/3
  Max_RX_Gain/1 -> Mux5/2
  Tx_Rx_Delayed/1 -> Mux5/1
  Divisor/1 -> Mux6/2, Relational1/2
  Up Sample1/1 -> Shift and lookup/1(In1)
  Max_Mic_Gain/1 -> Mux1/1
  Convert1/1 -> Scale2/1, Scale1/1, Scale3/1, Scale4/1
  Constant1/1 -> Convert1/1
  Scale2/1 -> Mux1/2
  Scale4/1 -> Mux1/5
  Scale3/1 -> Mux1/4
  Scale1/1 -> Mux1/3
  Relational1/1 -> Mux6/1
  Mux1/1 -> Mux5/3
  AddSub/1 -> Up Sample1/1
  Mux6/1 -> AddSub/1
  Constant3/1 -> AddSub/2

== system Xcvr_SSB_AM_2p5/Audio_and_Mode_Control/AGC_and_More/AGC Xilinx/Xabs ==
  In1 : Inport
  Mux : xbsIndex_r4/Mux  inputs=2  en=off  latency=0  precision=User Defined  arith_type=Unsigned  n_bits=16  bin_pt=15  quantization=Truncate  overflow=Wrap  dbl_ovrd=off  block_type=mux
      settings: block_version=9.2.00
  Negate : xbsIndex_r4/Negate  precision=User Defined  arith_type="Signed  (2's comp)"  n_bits=18  bin_pt=17  quantization=Truncate  overflow=Saturate  en=off  latency=0  dbl_ovrd=off  block_type=negate
      settings: block_version=9.2.00
  Slice : xbsIndex_r4/Slice  nbits=1  boolean_output=on  mode=Upper Bit Location + Width  bit1=0  base1=MSB of Input  bit0=0  base0=LSB of Input  dbl_ovrd=off  block_type=slice
      settings: block_version=9.2.00
  Out1 : Outport
  wires:
  Mux/1 -> Out1/1
  In1/1 -> Mux/2, Negate/1, Slice/1
  Negate/1 -> Mux/3
  Slice/1 -> Mux/1
